simulink model "Simple_Simulink_Try"  (R2018b)
settings: Solver=VariableStepDiscrete  StartTime=0.0  StopTime=inf  RelTol=1e-3
undefined symbols (not defined in the file): j
libraries: commdigbbndpm3 x2, commchan3 x1, commrandsrc3 x1, commeq2 x1, commlibv2 x1, commsink2 x1, commhdlmod x1, commsource2 x1
settings Model: Creator=nhj94  LastModifiedBy=nhj94
settings DataIOCC: LimitDataPoints=on  SaveOutput=off  SaveTime=off
settings OptimizationCC: BooleanDataType=off  DefaultParameterBehavior=Inlined  LocalBlockOutputs=off  LifeSpan=inf
settings DebuggingCC: AlgebraicLoopMsg=error  SingleTaskRateTransMsg=error  AllowSymbolicDim=off  SFUnexpectedBacktrackingDiag=warning  SFNoUnconditionalDefaultTransitionDiag=warning  SFExecutionAtInitializationDiag=none
settings SFSimCC: SimUseLocalCustomCode=off
settings RTWCC: RTWUseLocalCustomCode=off
settings CodeAppCC: StateflowObjectComments=on
settings GRTTargetCC: TargetLangStandard=C89/C90 (ANSI)  GeneratePreprocessorConditionals=Disable all
settings ConfigComp: CovMetricSettings=dw  CovHtmlReporting=on  CovSaveCumulativeToWorkspaceVar=on  CovSaveSingleToWorkspaceVar=on  CovExternalEMLEnable=off  CovSFcnEnable=off

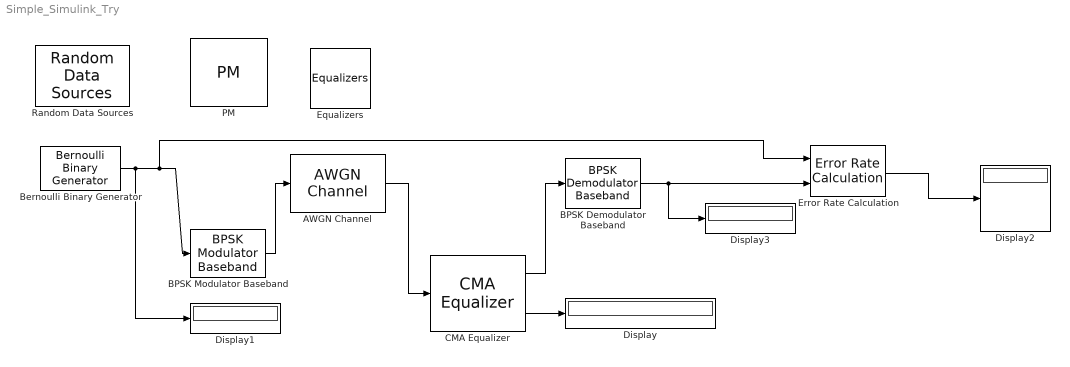
== system Simple_Simulink_Try ==
  AWGN Channel : commchan3/AWGN Channel  InputProcessing=Columns as channels (frame based)  seed=67  noiseMode="Signal to noise ratio  (Eb/No)"  EbNodB=10  EsNodB=10  SNRdB=10  bitsPerSym=1  Ps=1  Tsym=1  variance=1
  BPSK Demodulator Baseband : commdigbbndpm3/BPSK Demodulator Baseband  DecType=Hard decision  VarSource=Dialog  Variance=1  Ph=0  outDtype=Inherit via internal rule  derotateFactorWordLen=16  derotateFactorDataTypeStr=Inherit: Same word length as input  derotateFactorLastDataTypeStr=Inherit: Same word length as input
  BPSK Modulator Baseband : commdigbbndpm3/BPSK Modulator Baseband  Ph=0  outDtype=double  outWordLen=16  outUDDataType=sfix(16)  outFracLenMode=Best precision  outFracLen=15  outDataTypeStr=double  outLastDataTypeStr=double
  Bernoulli Binary Generator : commrandsrc3/Bernoulli Binary Generator  ProbabilityOfZero=0.5  SeedSource=Auto  Seed=0  SampleTime=1  SamplesPerFrame=1  OutputDataType=double  SimulateUsing=Interpreted execution
  CMA Equalizer : commeq2/CMA Equalizer  nTaps=4  nSamp=1  sigConst=[1+j -1+j -1-j 1-j]  stepSize=0.01  leakage=1  initWeights=[1 0 0 0]  outErr=on  outWeights=off
      settings: SourceProductName=Communications System Toolbox  SourceProductBaseCode=CM
  Display{,1..3} (4 alike) : Display
  Equalizers : commlibv2/Equalizers
      settings: SourceProductName=Communications System Toolbox  SourceProductBaseCode=CM
  Error Rate Calculation : commsink2/Error Rate Calculation  N=0  st_delay=0  cp_mode=Entire frame  subframe=[]  PMode=Port  WsName=ErrorVec  RsMode2=off  stop=off  numErr=100  maxBits=1e6
  PM : commhdlmod/PM
      settings: SourceProductName=Communications System Toolbox  SourceProductBaseCode=CM
  Random Data Sources : commsource2/Random Data Sources
      settings: SourceProductName=Communications System Toolbox  SourceProductBaseCode=CM
  wires:
  Bernoulli Binary Generator/1 -> Display1/1, Error Rate Calculation/1, BPSK Modulator Baseband/1
  BPSK Modulator Baseband/1 -> AWGN Channel/1
  BPSK Demodulator Baseband/1 -> Display3/1, Error Rate Calculation/2
  AWGN Channel/1 -> CMA Equalizer/1
  CMA Equalizer/1 -> BPSK Demodulator Baseband/1
  CMA Equalizer/2 -> Display/1
  Error Rate Calculation/1 -> Display2/1
